simulink model "lab5_adc"  (R2022b)
settings: Solver=VariableStepAuto  StartTime=0.0  StopTime=0.035  RelTol=1e-3
libraries: dspquant2 x2, dsparch4 x1, dspsigops x1
settings Model: Creator=12403  LastModifiedBy=12403

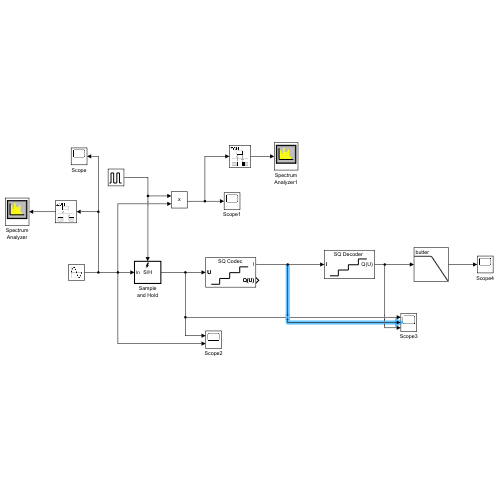
[thumbnail: Simulink's stored preview of the top-level diagram]
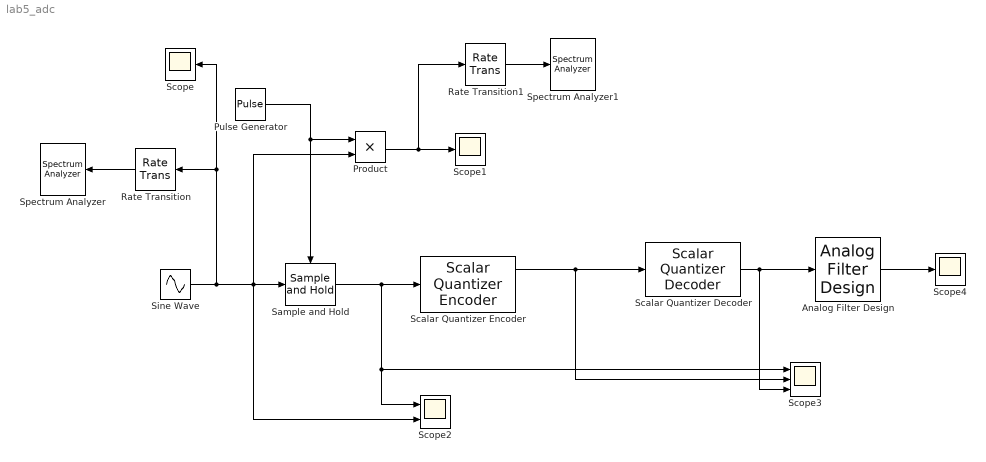
== system lab5_adc ==
  Analog Filter Design : dsparch4/Analog Filter Design  method=Butterworth  filttype=Lowpass  N=20  Wlo=2*pi*500  Whi=80  Rp=2  Rs=40
  Product : Product
  Pulse Generator : DiscretePulseGenerator  PulseType=Time based  Period=0.001/8  PulseWidth=50
  Rate Transition : RateTransition  OutPortSampleTime=1e-5
  Rate Transition1 : RateTransition  OutPortSampleTime=1e-5
  Sample and Hold : dspsigops/Sample and Hold  trig=Rising edge  initCond=0  latchinput=off
  Scalar Quantizer Decoder : dspquant2/Scalar Quantizer Decoder  invalidin=Clip  CBsource=Specify via dialog  codebook=[-1.75:0.5:1.75]  dataType=double  isSigned=on  wordLen=16  udDataType=sfix(16)  fracBitsMode=Best precision  numFracBits=11  OutDataTypeStr=double  LastOutDataTypeStr=double
  Scalar Quantizer Encoder : dspquant2/Scalar Quantizer Encoder  paramSrc=Specify via dialog  partType=Bounded  BBoundary=[-2:0.5:2]  UBoundary=[2:9]  SearchMethod=Binary  tieBreakRule=Choose the lower index  outQU=on  outQError=off  codebook=[-1.75:0.5:1.75]  outStatus=off  invalidin=Clip  idtype=int32  roundingMode=Floor  overflowMode=off
  Scope : Scope
  Scope1 : Scope
  Scope2 : Scope  NumInputPorts=2
  Scope3 : Scope  NumInputPorts=3
  Scope4 : Scope
  Sine Wave : Sin  Amplitude=2  Frequency=2*pi*500  SampleTime=0
  Spectrum Analyzer : SpectrumAnalyzer
  Spectrum Analyzer1 : SpectrumAnalyzer
  wires:
  Rate Transition/1 -> Spectrum Analyzer/1
  Sine Wave/1 -> Scope/1, Rate Transition/1, Product/2, Sample and Hold/1, Scope2/2
  Pulse Generator/1 -> Product/1, Sample and Hold/Trigger
  Product/1 -> Rate Transition1/1, Scope1/1
  Rate Transition1/1 -> Spectrum Analyzer1/1
  Sample and Hold/1 -> Scalar Quantizer Encoder/1, Scope3/1, Scope2/1
  Scalar Quantizer Encoder/1 -> Scalar Quantizer Decoder/1, Scope3/2
  Scalar Quantizer Decoder/1 -> Analog Filter Design/1, Scope3/3
  Analog Filter Design/1 -> Scope4/1
